simulink model "Control_sis_no_lineal_punto_operacion"  (R2016a)
settings: Solver=VariableStepAuto  StartTime=0.0  StopTime=30  RelTol=1e-3
values from neighbouring files (symbols this model uses):
  ki = kt(:,3:3)    [ejemplodiscretro.m]
undefined symbols (not defined in the file or in its folder): kp1, kp2
settings Model: Creator=Daniel  LastModifiedBy=Daniel

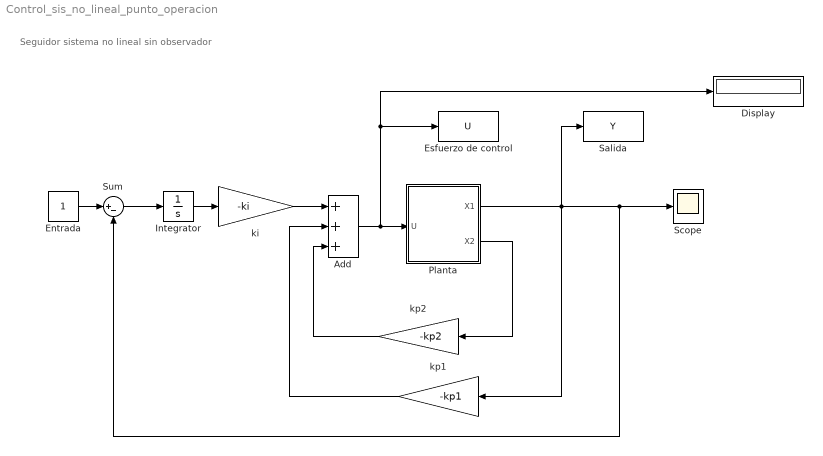
== system Control_sis_no_lineal_punto_operacion ==
  note: Seguidor sistema no lineal sin observador
  Add : Sum  Inputs=+++
  Display : Display
  Entrada : Constant
  Esfuerzo de control : ToWorkspace  VariableName=U  SaveFormat=Timeseries  SampleTime=-1
  Integrator : Integrator
  Planta : Subsystem
  Salida : ToWorkspace  VariableName=Y  SaveFormat=Timeseries  SampleTime=-1
  Scope : Scope
  Sum : Sum  Inputs=|+-
  ki : Gain  Gain=-ki
  kp1 : Gain  Gain=-kp1
  kp2 : Gain  Gain=-kp2
  wires:
  Add/1 -> Display/1, Esfuerzo de control/1, Planta/1(U)
  ki/1 -> Add/1
  Integrator/1 -> ki/1
  Sum/1 -> Integrator/1
  Entrada/1 -> Sum/1
  Planta/2(X2) -> kp2/1
  kp2/1 -> Add/3
  Planta/1(X1) -> Scope/1, Sum/2, Salida/1, kp1/1
  kp1/1 -> Add/2

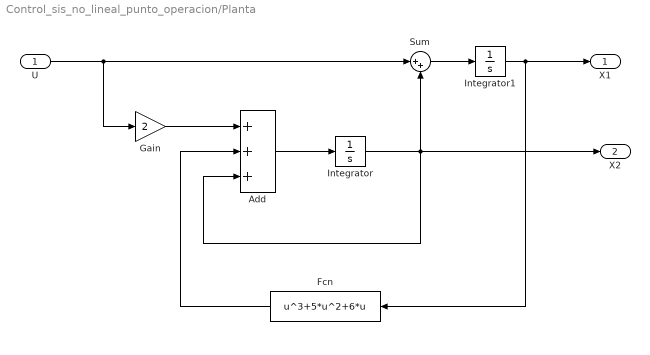
== system Control_sis_no_lineal_punto_operacion/Planta ==
  U : Inport
  Add : Sum  Inputs=+++
  Fcn : Fcn  Expr=u^3+5*u^2+6*u
  Gain : Gain  Gain=2
  Integrator : Integrator
  Integrator1 : Integrator
  Sum : Sum  Inputs=|++
  X1 : Outport
  X2 : Outport  Port=2
  wires:
  Integrator1/1 -> X1/1, Fcn/1
  Sum/1 -> Integrator1/1
  Integrator/1 -> X2/1, Sum/2, Add/3
  Add/1 -> Integrator/1
  Gain/1 -> Add/1
  Fcn/1 -> Add/2
  U/1 -> Gain/1, Sum/1
